simulink model "AutoPilot"  (R2018b)
settings: Solver=VariableStepAuto  StartTime=0.0  StopTime=1000  RelTol=1e-3
values from neighbouring files (symbols this model uses):
  a_phi1 = 2.87    [A2.m]    (also in prob3sim.m)
  a_phi2 = -0.65    [A2.m]    (also in prob3sim.m)
  d = 1.5    [A2.m]    (also in prob3sim.m)
  g = 9.81    [A2.m]    (also in prob3sim.m)
  k_dPhi = (2*z_rollDamp*omeg_NatRoll - a_phi1)/(a_phi2)    [A2.m]    (also in prob3sim.m)
  k_iPhi = 0    [A2.m]    (also in prob3sim.m)
  k_iPsi = omeg_NatPsi^2*(V_g/g)    [A2.m]    (also in prob3sim.m)
  k_pPhi = (z_aMax/e_rollMax)*sign(a_phi2)    [A2.m]    (also in prob3sim.m)
  k_pPsi = 2*z_courseDamp*omeg_NatPsi*(V_g/g)    [A2.m]    (also in prob3sim.m)
  V_g = V_a*(1000/(60*60))    (= 161.111111111)    [A2.m]    (also in prob3sim.m)
settings Model: Creator=Robert  LastModifiedBy=Robert

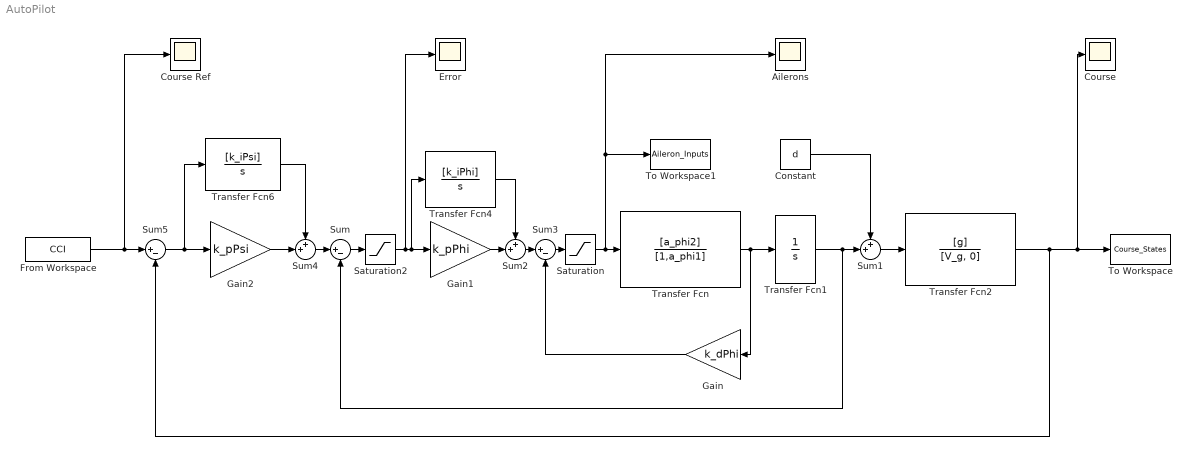
== system AutoPilot ==
  "Ailerons " : Scope
  Constant : Constant  Value=d
  "Course " : Scope
  "Course Ref " : Scope
  "Error " : Scope
  From Workspace : FromWorkspace  VariableName=CCI  SampleTime=0  Interpolate=off  OutputAfterFinalValue=Holding final value
  Gain : Gain  Gain=k_dPhi
  Gain1 : Gain  Gain=k_pPhi
  Gain2 : Gain  Gain=k_pPsi
  Saturation : Saturate  UpperLimit=30  LowerLimit=-30
  Saturation2 : Saturate  UpperLimit=15  LowerLimit=-15
  Sum : Sum  Inputs=|+-
  Sum1 : Sum  Inputs=++|
  Sum2 : Sum  Inputs=++|
  Sum3 : Sum  Inputs=|+-
  Sum4 : Sum  Inputs=++|
  Sum5 : Sum  Inputs=|+-
  To Workspace : ToWorkspace  VariableName=Course_States  SaveFormat=Timeseries  SampleTime=-1
  To Workspace1 : ToWorkspace  VariableName=Aileron_Inputs  SaveFormat=Timeseries  SampleTime=-1
  Transfer Fcn : TransferFcn  Numerator=[a_phi2]  Denominator=[1,a_phi1]
  Transfer Fcn1 : TransferFcn  Denominator=[1,0]
  Transfer Fcn2 : TransferFcn  Numerator=[g]  Denominator=[V_g, 0]
  Transfer Fcn4 : TransferFcn  Numerator=[k_iPhi]  Denominator=[1 0]
  Transfer Fcn6 : TransferFcn  Numerator=[k_iPsi]  Denominator=[1 0]
  wires:
  Transfer Fcn/1 -> Transfer Fcn1/1, Gain/1
  Transfer Fcn1/1 -> Sum/2, Sum1/2
  Constant/1 -> Sum1/1
  Sum1/1 -> Transfer Fcn2/1
  Sum2/1 -> Sum3/1
  Gain/1 -> Sum3/2
  Gain1/1 -> Sum2/2
  Transfer Fcn4/1 -> Sum2/1
  Sum/1 -> Saturation2/1
  Sum4/1 -> Sum/1
  Sum5/1 -> Transfer Fcn6/1, Gain2/1
  Transfer Fcn6/1 -> Sum4/1
  Gain2/1 -> Sum4/2
  Transfer Fcn2/1 -> "Course "/1, To Workspace/1, Sum5/2
  From Workspace/1 -> "Course Ref "/1, Sum5/1
  Sum3/1 -> Saturation/1
  Saturation/1 -> To Workspace1/1, "Ailerons "/1, Transfer Fcn/1
  Saturation2/1 -> "Error "/1, Transfer Fcn4/1, Gain1/1
